simulink library "aausat3_lib"  (Simulink 8.3)
settings: Solver=ode45  StartTime=0.0  StopTime=10.0  RelTol=1e-3
undefined symbols (not defined in the file or in its folder): A_wire_mt, albedo_wrapper, alpha_0_mt, bias_gyro, bias_mag, bias_sun, Cd, coil_dim, Dim, f_sample, G, heading_gyro, heading_mag, M_earth, M_moon, M_sun, magnitude, n_mt, noise_gyro, noise_mag, noise_sun, nr_sample_sun, otoquest, otoquest_with_pro, q_method, qmethod, redfac, refldata, s_freq_gyro, s_freq_mag, s_freq_sun, sigma_0_mt, solar_absorb_coeff, solar_m_flux, SVD_method, T_0_mt, theta_e, tilt_gyro, tilt_mag, Ts
undefined symbols (not defined in the file): Actuator_Duty_Cycle_coil, Actuator_Frequency_coil, Dimensions_coil, mean_refl, Number_of_Windings_coil, rho, sim_par, svd_weigth, Wire_Cross_Sectional_Area_coil, Wire_Resistivity_Base_Temperature_coil, Wire_Resistivity_coil, Wire_Resistivity_Temperature_Coefficient_coil
libraries: aausat3_lib x118, simulink_extras x3
(part 3 of 4)

== system aausat3_lib/Orbit and Ephemeris/SGP4 position ==
  JD : Inport
  TLE : Inport  Port=2
  Enable : EnablePort
  " S-Function" : S-Function  FunctionName=sgp4S  EnableBusSupport=off
  Demux : Demux  Outputs=12
  Demux1 : Demux  Outputs=[3 3]
  JD to Minutes : Gain  Gain=1440
  Mux : Mux  Inputs=2
  Mux1 : Mux  Inputs=12
  Sum : Sum  Inputs=-+|  SaturateOnIntegerOverflow=on  InputSameDT=on  OutDataTypeStr=Inherit: Same as first input
  "TLE -> JD converter" : aausat3_lib/Other Model Utilities/TLE -> JD converter  SystemSampleTime=-1
  "km -> m" : Gain  Gain=1000  SaturateOnIntegerOverflow=on  OutDataTypeStr=Inherit: Same as input  ParamDataTypeStr=Inherit: Same as input
  "km/s -> m/s" : Gain  Gain=1000  SaturateOnIntegerOverflow=on  OutDataTypeStr=Inherit: Same as input  ParamDataTypeStr=Inherit: Same as input
  Position (I) : Outport  InitialOutput=0
  Velocity (I) : Outport  Port=2  InitialOutput=0
  wires:
  JD/1 -> Sum/2
  "km -> m"/1 -> Position (I)/1
  "km/s -> m/s"/1 -> Velocity (I)/1
  Mux/1 -> " S-Function"/1
  " S-Function"/1 -> Demux1/1
  Demux1/2 -> "km/s -> m/s"/1
  Demux1/1 -> "km -> m"/1
  TLE/1 -> Demux/1
  Demux/2 -> Mux1/2
  Demux/3 -> Mux1/3
  Demux/4 -> Mux1/4
  Demux/5 -> Mux1/5
  Demux/6 -> Mux1/6
  Demux/7 -> Mux1/7
  Demux/8 -> Mux1/8
  Demux/9 -> Mux1/9
  Demux/10 -> Mux1/10
  Demux/11 -> Mux1/11
  Demux/12 -> Mux1/12
  Mux1/1 -> Mux/2
  Demux/1 -> "TLE -> JD converter"/1
  "TLE -> JD converter"/1 -> Mux1/1, Sum/1
  Sum/1 -> JD to Minutes/1
  JD to Minutes/1 -> Mux/1

== system aausat3_lib/Orbit and Ephemeris/TLE AAUSAT-II ==
  "Constant " : Constant  Value=[JulianDay,xndt2o,xndd6o,0,bstar,0,xincl,xnodeo,eo,omegao,xmo,xno]
  "TLE " : Outport
  wires:
  "Constant "/1 -> "TLE "/1

== system aausat3_lib/Orbit and Ephemeris/TLE Orsted ==
  "Constant " : Constant  Value=[JulianDay,xndt2o,xndd6o,0,bstar,0,xincl,xnodeo,eo,omegao,xmo,xno]
  "TLE " : Outport
  wires:
  "Constant "/1 -> "TLE "/1

== system aausat3_lib/Other Model Utilities/AAUSAT-II Animation ==
  SC position : Inport
  SC quaternion : Inport  Port=2
  SC veloc : Inport  Port=3
  sun vector(I) : Inport  Port=4
  Earth rotation : Inport  Port=5
  Mux3 : Mux  Inputs=5
  S-Function : S-Function  FunctionName=aausatanim  Parameters=Config  EnableBusSupport=off
  wires:
  SC veloc/1 -> Mux3/3
  Earth rotation/1 -> Mux3/5
  sun vector(I)/1 -> Mux3/4
  SC quaternion/1 -> Mux3/2
  SC position/1 -> Mux3/1
  Mux3/1 -> S-Function/1

== system aausat3_lib/Other Model Utilities/Exposed area ==
  quaternion : Inport
  vector : Inport  Port=2
  Product2 : Product  Multiplication=Matrix(*)  RndMeth=Zero
  Product3 : Product  Multiplication=Matrix(*)  RndMeth=Zero
  Product4 : Product  Multiplication=Matrix(*)  RndMeth=Zero
  Projection Matrix1 : Subsystem
  Satellite Area : aausat3_lib/Other Model Utilities/Satellite Area  SystemSampleTime=-1
  To unit vector : aausat3_lib/Math Utilities/Vector operations/To unit vector  SystemSampleTime=-1
  Vector rotation by q : aausat3_lib/Math Utilities/Quaternion operations/Vector rotation by q  SystemSampleTime=-1
  x : Constant  Value=[dim_sat_area(1) 0 0]'
  y : Constant  Value=[0 dim_sat_area(2) 0]'
  z : Constant  Value=[0 0 dim_sat_area(3)]'
  exposed area : Outport
  wires:
  To unit vector/1 -> Vector rotation by q/2
  vector/1 -> To unit vector/1
  quaternion/1 -> Vector rotation by q/1
  Projection Matrix1/1(P matrix) -> Product2/1, Product4/1, Product3/1
  x/1 -> Product2/2
  y/1 -> Product4/2
  z/1 -> Product3/2
  Product2/1 -> Satellite Area/1
  Product4/1 -> Satellite Area/2
  Product3/1 -> Satellite Area/3
  Vector rotation by q/1 -> Projection Matrix1/1(n-vector)
  Satellite Area/1 -> exposed area/1

== system aausat3_lib/Other Model Utilities/Geocentric to  Geodetic Latitude ==
  lambda : Inport
  dist to body : Inport  Port=2
  Constant : Constant  Value=R
  Constant1 : Constant  Value=R
  Gain : Gain  Gain=pi/180
  Gain1 : Gain  Gain=180/pi
  Sum1 : Sum  Inputs=|-+
  Trigonometric Function : Trigonometry  Operator=tan
  alt : Subsystem
  delt_mu : Subsystem
  delta_lambda : Subsystem
  denom : Subsystem
  e : Subsystem
  e^4 : Subsystem
  l_point : Subsystem
  mu_alpha : Subsystem
  r_alpha : Subsystem
  rho_alpha : Subsystem
  square e : Subsystem
  square e1 : Subsystem
  x_alpha : Subsystem
  mu : Outport
  wires:
  Gain1/1 -> mu/1
  Gain/1 -> Trigonometric Function/1, mu_alpha/4(lambda), delta_lambda/2(lambda), r_alpha/1(lambda)
  dist to body/1 -> l_point/1(dist to body)
  lambda/1 -> Gain/1
  e/1(e) -> square e/1(e), x_alpha/3(e), e^4/1(e), mu_alpha/3(e)
  square e/1(e^2) -> x_alpha/4(e^2)
  Constant/1 -> square e1/1(R), x_alpha/1(R)
  square e1/1(R^2) -> mu_alpha/1(R^2)
  mu_alpha/1(mu_alpha) -> delta_lambda/1(mu_alpha), denom/1(mu_alpha), Sum1/2
  x_alpha/1(x_alpha) -> mu_alpha/2(x_alpha), r_alpha/2(x_alpha)
  Trigonometric Function/1 -> x_alpha/2(t_lat)  "t_lat"
  r_alpha/1(r_alpha) -> l_point/2(r_alpha)
  delta_lambda/1(delta_lambda) -> alt/2(delta_lambda), delt_mu/3(delta_lambda)
  l_point/1(l_point) -> alt/1(l_point), delt_mu/1(l_point)
  e^4/1(eps) -> denom/2(eps), rho_alpha/3(eps)
  denom/1(denom) -> rho_alpha/2(denom)
  alt/1(alt) -> delt_mu/2(alt)
  rho_alpha/1(rho_alpha) -> delt_mu/4(rho_alpha)
  delt_mu/1(delt_mu) -> Sum1/1
  Sum1/1 -> Gain1/1
  Constant1/1 -> rho_alpha/1(R)

== system aausat3_lib/Other Model Utilities/Geodetic to  Geocentric Latitude ==
  mu : Inport
  h : Inport  Port=2
  Constant : Constant  Value=F
  Demux : Demux  Outputs=2
  Mux : Mux  Inputs=2
  Mux1 : Mux  Inputs=2
  Product1 : Product  RndMeth=Zero
  Product2 : Product  Inputs=3  RndMeth=Zero
  Product3 : Product  RndMeth=Zero
  Radius at Geocentric Latitude : Subsystem  mask(Radius at Geocentric Latitude){units=Metric (MKS), ptype=Custom, F=F, R=R}
      mask prompts: ptype "Planet model:"; F "Flattening:"; R "Equatorial radius of planet:"
      mask help: Estimate radius of ellipsoid planet at geocentric latitude.
      mask init:
      | aeroicon('aeroblklla')
      mask Help: eval('asbhelp');
      mask TypeOptions units: Metric (MKS) | English
      mask TypeOptions ptype: Custom | Earth (WGS84)
      mask Callback ptype: aeroicon('aeroblklla')
      mask Display:
      | port_label('input',1,'\lambda_s','texmode','on')
      | port_label('output',1,'r_s','texmode','on')
  Sum : Sum  Inputs=-+
  Sum1 : Sum  Inputs=|++
  Trigonometric Function1 : Trigonometry  Operator=tan
  Trigonometric Function2 : Trigonometry  Operator=atan2
  Trigonometric Function3 : Trigonometry  Operator=atan2
  f : Constant
  rad->deg : Gain  Gain=180/pi
  rad->deg1 : Gain  Gain=180/pi
  sincos : Trigonometry  Operator=sincos
  sincos1 : Trigonometry  Operator=sincos
  lambda : Outport
  wires:
  rad->deg1/1 -> Radius at Geocentric Latitude/1(lambda_s)
  mu/1 -> sincos1/1, Trigonometric Function1/1
  Constant/1 -> Sum/1
  f/1 -> Trigonometric Function2/2, Sum/2
  Product2/1 -> Trigonometric Function2/1
  Sum/1 -> Product2/3, Product2/2
  Trigonometric Function2/1 -> sincos/1, rad->deg1/1
  Trigonometric Function1/1 -> Product2/1
  Radius at Geocentric Latitude/1(r_s) -> Product1/1
  rad->deg/1 -> lambda/1
  sincos1/1 -> Mux/1
  h/1 -> Product3/1
  sincos1/2 -> Mux/2
  sincos/1 -> Mux1/1
  sincos/2 -> Mux1/2
  Mux/1 -> Product3/2
  Mux1/1 -> Product1/2
  Product3/1 -> Sum1/1
  Product1/1 -> Sum1/2
  Trigonometric Function3/1 -> rad->deg/1
  Sum1/1 -> Demux/1
  Demux/1 -> Trigonometric Function3/1
  Demux/2 -> Trigonometric Function3/2

== system aausat3_lib/Other Model Utilities/Randome 3D Vector ==
  Demux : Demux  Outputs=3
  Divide : Product  Inputs=*/
  Math Function : Math  Operator=square  SaturateOnIntegerOverflow=on
  Math Function1 : Math  Operator=square  SaturateOnIntegerOverflow=on
  Math Function2 : Math  Operator=square  SaturateOnIntegerOverflow=on
  Math Function3 : Math  Operator=sqrt  SaturateOnIntegerOverflow=on
  Random Number : RandomNumber  Mean=mean  Variance=[var,0,0]  Seed=seed(1)
  Random Number1 : RandomNumber  Mean=mean  Variance=[0,var,0]  Seed=seed(2)
  Random Number2 : RandomNumber  Mean=mean  Variance=[0,0,var]  Seed=seed(3)
  Sum : Sum  Inputs=+++
  Sum1 : Sum  Inputs=+++
  Sum2 : Sum  Inputs=+++
  Rand_vec : Outport
  wires:
  Divide/1 -> Rand_vec/1
  Sum2/1 -> Math Function3/1
  Demux/3 -> Sum2/3
  Demux/2 -> Sum2/2
  Demux/1 -> Sum2/1
  Sum/1 -> Demux/1
  Sum1/1 -> Divide/1
  Math Function3/1 -> Divide/2
  Random Number2/1 -> Sum1/3, Math Function2/1
  Random Number1/1 -> Sum1/2, Math Function1/1
  Random Number/1 -> Sum1/1, Math Function/1
  Math Function2/1 -> Sum/3
  Math Function1/1 -> Sum/2
  Math Function/1 -> Sum/1

== system aausat3_lib/Other Model Utilities/SC ECI to geodetic position converter ==
  Simulation time  t(JD) : Inport
  Spacecraft position R_sc(I) : Inport  Port=2
  Cartesian to Spherical : simulink_extras/Transformations/Cartesian to Spherical  SystemSampleTime=-1
  Demux1 : Demux  Outputs=3
  ECI->ECEF quaternion : aausat3_lib/Orbit and Ephemeris/ECI->ECEF quaternion  SystemSampleTime=-1
  Earth radius WGS84 : Fcn  Expr=sqrt(((a^2*cos(u(1)))^2+(b^2*sin(u(1)))^2)/((a*cos(u(1)))^2+(b*sin(u(1)))^2))
  Eccentricity : Constant  Value=sqrt(a^2-b^2)/a
  Geocentric to  Geodetic Latitude : aausat3_lib/Other Model Utilities/Geocentric to  Geodetic Latitude  SystemSampleTime=-1
  Geodetic elevation : Fcn  Expr=(u(4)*cos(pi/180*u(3)-pi/180*u(5))-1/u(1))/1000-u(2)
  Mux : Mux  Inputs=2
  Mux1 : Mux  Inputs=5
  N : Fcn  Expr=(1-u(1)^2*sin(u(2))^2)^(-1/2)
  Vector rotation by q : aausat3_lib/Math Utilities/Quaternion operations/Vector rotation by q  SystemSampleTime=-1
  convert to  geocentric latitude : Fcn  Expr=(90-180/pi*u(1))
  convert to  geocentric longitude : Fcn  Expr=180/pi*u(1)
  Geodetic elevation (km) : Outport
  Geodetic longitude  (degree) : Outport  Port=2
  Geodetic latitude  (degree) : Outport  Port=3
  wires:
  Spacecraft position R_sc(I)/1 -> Vector rotation by q/2
  Vector rotation by q/1 -> Demux1/1
  Demux1/1 -> Cartesian to Spherical/1
  Demux1/2 -> Cartesian to Spherical/2
  Demux1/3 -> Cartesian to Spherical/3
  Cartesian to Spherical/1 -> Geocentric to  Geodetic Latitude/2, Mux1/4
  Cartesian to Spherical/2 -> convert to  geocentric longitude/1
  Cartesian to Spherical/3 -> convert to  geocentric latitude/1
  Simulation time  t(JD)/1 -> ECI->ECEF quaternion/1
  ECI->ECEF quaternion/1 -> Vector rotation by q/1
  convert to  geocentric latitude/1 -> Geocentric to  Geodetic Latitude/1, Mux1/5
  convert to  geocentric longitude/1 -> Geodetic longitude  (degree)/1
  Geocentric to  Geodetic Latitude/1 -> Geodetic latitude  (degree)/1, Earth radius WGS84/1, Mux/2, Mux1/3
  Mux/1 -> N/1
  Eccentricity/1 -> Mux/1
  Mux1/1 -> Geodetic elevation/1
  Earth radius WGS84/1 -> Mux1/2
  N/1 -> Mux1/1
  Geodetic elevation/1 -> Geodetic elevation (km)/1

== system aausat3_lib/Other Model Utilities/Satellite Area ==
  px : Inport
  py : Inport  Port=2
  pz : Inport  Port=3
  Cross Product : aausat3_lib/Math Utilities/Vector operations/Cross Product  SystemSampleTime=-1
  Cross Product1 : aausat3_lib/Math Utilities/Vector operations/Cross Product  SystemSampleTime=-1
  Cross Product2 : aausat3_lib/Math Utilities/Vector operations/Cross Product  SystemSampleTime=-1
  Dot Product : DotProduct  InputSameDT=on  OutDataTypeStr=Inherit: Inherit via internal rule
  Dot Product1 : DotProduct  InputSameDT=on  OutDataTypeStr=Inherit: Inherit via internal rule
  Dot Product2 : DotProduct  InputSameDT=on  OutDataTypeStr=Inherit: Inherit via internal rule
  Sum : Sum  Inputs=+|+|+
  inv1 : Math  Operator=sqrt  SaturateOnIntegerOverflow=on
  inv2 : Math  Operator=sqrt  SaturateOnIntegerOverflow=on
  inv3 : Math  Operator=sqrt  SaturateOnIntegerOverflow=on
  area_sat : Outport
  wires:
  Dot Product/1 -> inv1/1
  Cross Product/1 -> Dot Product/2, Dot Product/1
  px/1 -> Cross Product/1, Cross Product1/1
  inv1/1 -> Sum/1
  py/1 -> Cross Product/2, Cross Product2/1
  Dot Product1/1 -> inv2/1
  Cross Product1/1 -> Dot Product1/1, Dot Product1/2
  Dot Product2/1 -> inv3/1
  Cross Product2/1 -> Dot Product2/2, Dot Product2/1
  pz/1 -> Cross Product1/2, Cross Product2/2
  inv2/1 -> Sum/2
  inv3/1 -> Sum/3
  Sum/1 -> area_sat/1

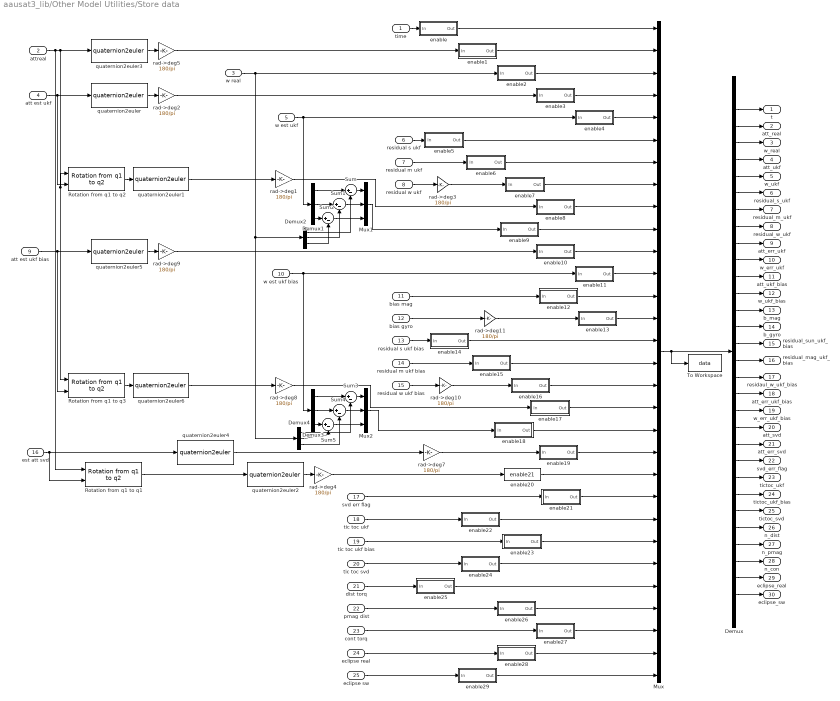
== system aausat3_lib/Other Model Utilities/Store data ==
  time : Inport
  attreal : Inport  Port=2
  w real : Inport  Port=3
  att est ukf : Inport  Port=4
  w est ukf : Inport  Port=5
  residual s ukf : Inport  Port=6
  residual m ukf : Inport  Port=7
  residual w ukf : Inport  Port=8
  att est ukf bias : Inport  Port=9
  w est ukf bias : Inport  Port=10
  bias mag : Inport  Port=11
  bias gyro : Inport  Port=12
  residual s ukf bias : Inport  Port=13
  residual m ukf bias : Inport  Port=14
  residual w ukf bias : Inport  Port=15
  est att svd : Inport  Port=16
  svd err flag : Inport  Port=17
  tic toc ukf : Inport  Port=18
  tic toc ukf bias : Inport  Port=19
  tic toc svd : Inport  Port=20
  dist torq : Inport  Port=21
  pmag dist : Inport  Port=22
  cont torq : Inport  Port=23
  eclipse real : Inport  Port=24
  eclipse sw : Inport  Port=25
  Demux : Demux  Outputs=30
  Demux{1..4} (4 alike) : Demux  Outputs=3
  Mux : Mux  Inputs=30
  Mux1 : Mux  Inputs=3
  Mux2 : Mux  Inputs=3
  Rotation from q1 to q1 : aausat3_lib/Math Utilities/Quaternion operations/Rotation from q1 to q2  SystemSampleTime=-1
  Rotation from q1 to q2 : aausat3_lib/Math Utilities/Quaternion operations/Rotation from q1 to q2  SystemSampleTime=-1
  Rotation from q1 to q3 : aausat3_lib/Math Utilities/Quaternion operations/Rotation from q1 to q2  SystemSampleTime=-1
  Sum{,1..5} (6 alike) : Sum  Inputs=|+-
  To Workspace : ToWorkspace  VariableName=data  SampleTime=1/f_sample
  enable : Subsystem  mask{enable_signal=enable_t}
      mask prompts: enable_signal "Signal name:"
  enable1 : Subsystem  mask{enable_signal=enable_att}
      mask prompts: enable_signal "Signal name:"
  enable10 : Subsystem  mask{enable_signal=enable_att_ukf_bias}
      mask prompts: enable_signal "Signal name:"
  enable11 : Subsystem  mask{enable_signal=enable_w_ukf_bias}
      mask prompts: enable_signal "Signal name:"
  enable12 : Subsystem  mask{enable_signal=enable_b_mag}
      mask prompts: enable_signal "Signal name:"
  enable13 : Subsystem  mask{enable_signal=enable_b_gyro}
      mask prompts: enable_signal "Signal name:"
  enable14 : Subsystem  mask{enable_signal=enable_r_sun_ukf_bias}
      mask prompts: enable_signal "Signal name:"
  enable15 : Subsystem  mask{enable_signal=enable_r_mag_ukf_bias}
      mask prompts: enable_signal "Signal name:"
  enable16 : Subsystem  mask{enable_signal=enable_r_w_ukf_bias}
      mask prompts: enable_signal "Signal name:"
  enable17 : Subsystem  mask{enable_signal=enable_eia_ukf_bias}
      mask prompts: enable_signal "Signal name:"
  enable18 : Subsystem  mask{enable_signal=enable_eiw_ukf_bias}
      mask prompts: enable_signal "Signal name:"
  enable19 : Subsystem  mask{enable_signal=enable_att_svd}
      mask prompts: enable_signal "Signal name:"
  enable2 : Subsystem  mask{enable_signal=enable_w}
      mask prompts: enable_signal "Signal name:"
  enable20 : aausat3_lib/Other Model Utilities/Store data/enable21  SystemSampleTime=-1  enable_signal=enable_svd_att_err
  enable21 : Subsystem  mask{enable_signal=enable_svd_err}
      mask prompts: enable_signal "Signal name:"
  enable22 : Subsystem  mask{enable_signal=enable_tictoc}
      mask prompts: enable_signal "Signal name:"
  enable23 : Subsystem  mask{enable_signal=enable_tictoc_ukf_bias}
      mask prompts: enable_signal "Signal name:"
  enable24 : Subsystem  mask{enable_signal=enable_tictoc_svd}
      mask prompts: enable_signal "Signal name:"
  enable25 : Subsystem  mask{enable_signal=enable_n_dist}
      mask prompts: enable_signal "Signal name:"
  enable26 : Subsystem  mask{enable_signal=enable_n_pmag}
      mask prompts: enable_signal "Signal name:"
  enable27 : Subsystem  mask{enable_signal=enable_n_con}
      mask prompts: enable_signal "Signal name:"
  enable28 : Subsystem  mask{enable_signal=enable_eclip_real}
      mask prompts: enable_signal "Signal name:"
  enable29 : Subsystem  mask{enable_signal=enable_eclip_sw}
      mask prompts: enable_signal "Signal name:"
  enable3 : Subsystem  mask{enable_signal=enable_att_ukf}
      mask prompts: enable_signal "Signal name:"
  enable4 : Subsystem  mask{enable_signal=enable_w_ukf}
      mask prompts: enable_signal "Signal name:"
  enable5 : Subsystem  mask{enable_signal=enable_r_sun}
      mask prompts: enable_signal "Signal name:"
  enable6 : Subsystem  mask{enable_signal=enable_r_mag}
      mask prompts: enable_signal "Signal name:"
  enable7 : Subsystem  mask{enable_signal=enable_r_w}
      mask prompts: enable_signal "Signal name:"
  enable8 : Subsystem  mask{enable_signal=enable_eia}
      mask prompts: enable_signal "Signal name:"
  enable9 : Subsystem  mask{enable_signal=enable_eiw}
      mask prompts: enable_signal "Signal name:"
  quaternion2euler{,1..6} (7 alike) : aausat3_lib/Math Utilities/Quaternion operations/quaternion2euler  SystemSampleTime=-1
  rad->deg{1..5,7..11} (10 alike) : Gain  Gain=180/pi
  t : Outport
  att_real : Outport  Port=2
  w_real : Outport  Port=3
  att_ukf : Outport  Port=4
  w_ukf : Outport  Port=5
  residual_s_ukf : Outport  Port=6
  residual_m_ukf : Outport  Port=7
  residual_w_ukf : Outport  Port=8
  att_err_ukf : Outport  Port=9
  w_err_ukf : Outport  Port=10
  att_ukf_bias : Outport  Port=11
  w_ukf_bias : Outport  Port=12
  b_mag : Outport  Port=13
  b_gyro : Outport  Port=14
  residual_sun_ukf_bias : Outport  Port=15
  residual_mag_ukf_bias : Outport  Port=16
  residaul_w_ukf_bias : Outport  Port=17
  att_err_ukf_bias : Outport  Port=18
  w_err_ukf_bias : Outport  Port=19
  att_svd : Outport  Port=20
  att_err_svd : Outport  Port=21
  svd_err_flag : Outport  Port=22
  tictoc_ukf : Outport  Port=23
  tictoc_ukf_bias : Outport  Port=24
  tictoc_svd : Outport  Port=25
  n_dist : Outport  Port=26
  n_pmag : Outport  Port=27
  n_con : Outport  Port=28
  eclipse_real : Outport  Port=29
  eclipse_sw : Outport  Port=30
  wires:
  Demux/22 -> svd_err_flag/1
  Demux/25 -> tictoc_svd/1
  Demux/26 -> n_dist/1
  Demux/30 -> eclipse_sw/1
  Demux/29 -> eclipse_real/1
  Demux/28 -> n_con/1
  Demux/27 -> n_pmag/1
  Demux/24 -> tictoc_ukf_bias/1
  Demux/23 -> tictoc_ukf/1
  enable21/1(Out) -> Mux/22
  svd err flag/1 -> enable21/1(In)
  enable24/1(Out) -> Mux/25
  tic toc svd/1 -> enable24/1(In)
  enable29/1(Out) -> Mux/30
  eclipse sw/1 -> enable29/1(In)
  enable25/1(Out) -> Mux/26
  enable26/1(Out) -> Mux/27
  enable28/1(Out) -> Mux/29
  dist torq/1 -> enable25/1(In)
  pmag dist/1 -> enable26/1(In)
  cont torq/1 -> enable27/1(In)
  eclipse real/1 -> enable28/1(In)
  enable23/1(Out) -> Mux/24
  tic toc ukf bias/1 -> enable23/1(In)
  enable22/1(Out) -> Mux/23
  tic toc ukf/1 -> enable22/1(In)
  enable27/1(Out) -> Mux/28
  Demux/21 -> att_err_svd/1
  Demux/20 -> att_svd/1
  Demux/19 -> w_err_ukf_bias/1
  Demux/18 -> att_err_ukf_bias/1
  Demux/17 -> residaul_w_ukf_bias/1
  Demux/16 -> residual_mag_ukf_bias/1
  Demux/15 -> residual_sun_ukf_bias/1
  Demux/14 -> b_gyro/1
  Demux/13 -> b_mag/1
  Demux/12 -> w_ukf_bias/1
  Demux/11 -> att_ukf_bias/1
  Demux/10 -> w_err_ukf/1
  Demux/9 -> att_err_ukf/1
  Demux/8 -> residual_w_ukf/1
  Demux/7 -> residual_m_ukf/1
  Demux/6 -> residual_s_ukf/1
  Demux/5 -> w_ukf/1
  Demux/4 -> att_ukf/1
  Demux/3 -> w_real/1
  Demux/2 -> att_real/1
  Demux/1 -> t/1
  enable5/1(Out) -> Mux/6
  enable6/1(Out) -> Mux/7
  enable7/1(Out) -> Mux/8
  enable8/1(Out) -> Mux/9
  enable9/1(Out) -> Mux/10
  enable10/1(Out) -> Mux/11
  enable11/1(Out) -> Mux/12
  enable12/1(Out) -> Mux/13
  enable13/1(Out) -> Mux/14
  enable15/1(Out) -> Mux/16
  enable14/1(Out) -> Mux/15
  enable16/1(Out) -> Mux/17
  enable17/1(Out) -> Mux/18
  enable18/1(Out) -> Mux/19
  enable19/1(Out) -> Mux/20
  Demux4/3 -> Sum4/2
  Demux4/2 -> Sum5/2
  enable20/1 -> Mux/21
  enable4/1(Out) -> Mux/5
  enable3/1(Out) -> Mux/4
  enable2/1(Out) -> Mux/3
  enable1/1(Out) -> Mux/2
  enable/1(Out) -> Mux/1
  residual s ukf bias/1 -> enable14/1(In)
  w est ukf bias/1 -> enable11/1(In), Demux3/1
  bias mag/1 -> enable12/1(In)
  residual m ukf bias/1 -> enable15/1(In)
  Demux3/3 -> Sum5/1
  Demux4/1 -> Sum3/2
  Sum4/1 -> Mux2/2
  Sum5/1 -> Mux2/3
  Sum3/1 -> Mux2/1
  Demux3/2 -> Sum4/1
  Demux3/1 -> Sum3/1
  bias gyro/1 -> rad->deg11/1
  rad->deg11/1 -> enable13/1(In)
  quaternion2euler6/1 -> rad->deg8/1
  quaternion2euler5/1 -> rad->deg9/1
  att est ukf bias/1 -> Rotation from q1 to q3/2, quaternion2euler5/1
  Rotation from q1 to q3/1 -> quaternion2euler6/1
  residual w ukf bias/1 -> rad->deg10/1
  rad->deg10/1 -> enable16/1(In)
  rad->deg9/1 -> enable10/1(In)
  rad->deg8/1 -> enable17/1(In)
  Mux2/1 -> enable18/1(In)
  rad->deg7/1 -> enable19/1(In)
  quaternion2euler4/1 -> rad->deg7/1
  Mux/1 -> To Workspace/1, Demux/1
  time/1 -> enable/1(In)
  w real/1 -> Demux4/1, Demux2/1, enable2/1(In)
  w est ukf/1 -> enable4/1(In), Demux1/1
  residual s ukf/1 -> enable5/1(In)
  residual m ukf/1 -> enable6/1(In)
  est att svd/1 -> quaternion2euler4/1, Rotation from q1 to q1/2
  Demux1/3 -> Sum2/1
  Demux2/3 -> Sum2/2
  Demux2/2 -> Sum1/2
  Demux2/1 -> Sum/2
  Sum1/1 -> Mux1/2
  Sum2/1 -> Mux1/3
  Sum/1 -> Mux1/1
  Demux1/2 -> Sum1/1
  Demux1/1 -> Sum/1
  quaternion2euler2/1 -> rad->deg4/1
  Rotation from q1 to q1/1 -> quaternion2euler2/1
  quaternion2euler3/1 -> rad->deg5/1
  attreal/1 -> Rotation from q1 to q3/1, Rotation from q1 to q2/1, quaternion2euler3/1, Rotation from q1 to q1/1
  quaternion2euler1/1 -> rad->deg1/1
  quaternion2euler/1 -> rad->deg2/1
  att est ukf/1 -> Rotation from q1 to q2/2, quaternion2euler/1
  Rotation from q1 to q2/1 -> quaternion2euler1/1
  rad->deg5/1 -> enable1/1(In)
  residual w ukf/1 -> rad->deg3/1
  rad->deg3/1 -> enable7/1(In)
  rad->deg2/1 -> enable3/1(In)
  rad->deg1/1 -> enable8/1(In)
  Mux1/1 -> enable9/1(In)
  rad->deg4/1 -> enable20/1

== system aausat3_lib/Other Model Utilities/TLE -> JD converter ==
  TLE (Epoch time) : Inport
  Add century : Constant  Value=1900
  Add century1 : Constant  Value=2000
  Gain1 : Gain  Gain=1/1000
  Gain2 : Gain  Gain=1/1000
  Gain3 : Gain  Gain=1000
  Sum1 : Sum  Inputs=++|
  Sum3 : Sum  Inputs=++|
  Sum4 : Sum  Inputs=++-
  Sum5 : Sum  Inputs=|+-
  calculate JD for given year  at 1. jan time 00.00 : Fcn  Expr=367*u(1)-floor(7*(u(1)+floor((1+9)/12))/4)+floor(275*1/9)+1+1721013.5+0/24
  extract year : Rounding
  substract 1 day : Constant
  year 1950-1999 or  2000-2049? : Switch  Threshold=50
  JD : Outport
  wires:
  Add century/1 -> Sum3/1
  Gain2/1 -> Sum3/2, year 1950-1999 or  2000-2049?/2
  TLE (Epoch time)/1 -> Gain2/1, Gain1/1
  extract year/1 -> Sum5/2, calculate JD for given year  at 1. jan time 00.00/1
  calculate JD for given year  at 1. jan time 00.00/1 -> Sum4/2
  Sum5/1 -> Gain3/1
  Sum4/1 -> JD/1
  Gain3/1 -> Sum4/1
  substract 1 day/1 -> Sum4/3
  Add century1/1 -> Sum1/1
  Gain1/1 -> Sum1/2
  year 1950-1999 or  2000-2049?/1 -> extract year/1, Sum5/1
  Sum1/1 -> year 1950-1999 or  2000-2049?/3
  Sum3/1 -> year 1950-1999 or  2000-2049?/1

== system aausat3_lib/Sensor Emulation/Gyroscopes ==
  Omega_S : Inport
  Bias1 : Constant  Value=bias_gyro
  Cartesian to Spherical : aausat3_lib/Sensor Emulation/Sun sensors/Cartesian to Spherical  SystemSampleTime=-1
  Demux1 : Demux  Outputs=3
  Demux2 : Demux  Outputs=3
  Demux3 : Demux  Outputs=3
  Mux1 : Mux  Inputs=3
  Mux2 : Mux  Inputs=3
  Noise1 : RandomNumber  Variance=((pi/180)*noise_gyro)^2  Seed=1  SampleTime=0.1
  Noise2 : RandomNumber  Variance=((pi/180)*noise_gyro)^2  Seed=999  SampleTime=0.1
  Noise3 : RandomNumber  Variance=((pi/180)*noise_gyro)^2  Seed=46945  SampleTime=0.1
  Spherical to Cartesian : aausat3_lib/Sensor Emulation/Sun sensors/Spherical to Cartesian  SystemSampleTime=-1
  Sum1 : Sum  Inputs=|++
  Sum3 : Sum  Inputs=+++
  Sum6 : Sum  Inputs=+++
  Sum7 : Sum  Inputs=+++
  Sum8 : Sum  Inputs=|++
  Zero-Order Hold : ZeroOrderHold  SampleTime=1/s_freq_gyro
  "deg -> rad" : Gain  Gain=pi/180
  "deg -> rad1" : Gain  Gain=pi/180
  "deg -> rad2" : Gain  Gain=pi/180
  displacement : Constant  Value=heading_gyro
  displacement1 : Constant  Value=tilt_gyro
  Omega_S_meas : Outport
  wires:
  Noise1/1 -> Sum6/3
  "deg -> rad2"/1 -> Sum8/2
  displacement1/1 -> "deg -> rad2"/1
  "deg -> rad1"/1 -> Sum1/2
  displacement/1 -> "deg -> rad1"/1
  "deg -> rad"/1 -> Demux3/1
  Bias1/1 -> "deg -> rad"/1
  Noise2/1 -> Sum7/3
  Noise3/1 -> Sum3/3
  Zero-Order Hold/1 -> Omega_S_meas/1
  Omega_S/1 -> Demux1/1
  Demux1/3 -> Sum3/2
  Demux1/2 -> Sum7/2
  Demux1/1 -> Sum6/2
  Sum3/1 -> Mux1/3
  Sum7/1 -> Mux1/2
  Sum6/1 -> Mux1/1
  Demux2/1 -> Cartesian to Spherical/1
  Demux2/2 -> Cartesian to Spherical/2
  Demux2/3 -> Cartesian to Spherical/3
  Spherical to Cartesian/1 -> Mux2/1
  Spherical to Cartesian/2 -> Mux2/2
  Spherical to Cartesian/3 -> Mux2/3
  Cartesian to Spherical/1 -> Spherical to Cartesian/1
  Cartesian to Spherical/2 -> Sum1/1
  Sum1/1 -> Spherical to Cartesian/2
  Sum8/1 -> Spherical to Cartesian/3
  Cartesian to Spherical/3 -> Sum8/1
  Mux1/1 -> Demux2/1
  Mux2/1 -> Zero-Order Hold/1
  Demux3/1 -> Sum6/1
  Demux3/2 -> Sum7/1
  Demux3/3 -> Sum3/1

== system aausat3_lib/Sensor Emulation/Magnetometers ==
  q_I_S : Inport
  Mag_I : Inport  Port=2
  Bias : Constant  Value=bias_mag
  Cartesian to Spherical : aausat3_lib/Sensor Emulation/Sun sensors/Cartesian to Spherical  SystemSampleTime=-1
  Demux : Demux  Outputs=3
  Demux1 : Demux  Outputs=3
  Demux2 : Demux  Outputs=3
  Mux : Mux  Inputs=3
  Mux2 : Mux  Inputs=3
  Noise1 : RandomNumber  Variance=((pi/180)*noise_mag)^2  Seed=23771  SampleTime=0.1
  Noise2 : RandomNumber  Variance=((pi/180)*noise_mag)^2  Seed=5000  SampleTime=0.1
  Spherical to Cartesian : aausat3_lib/Sensor Emulation/Sun sensors/Spherical to Cartesian  SystemSampleTime=-1
  Sum : Sum  Inputs=++|
  Sum1 : Sum  Inputs=+++
  Sum2 : Sum  Inputs=+++
  Sum4 : Sum  Inputs=++|
  Sum5 : Sum  Inputs=++|
  Vector rotation by q : Subsystem
  Zero-Order Hold : ZeroOrderHold  SampleTime=1/s_freq_mag
  "[nT] -> [T]" : Gain  Gain=10^(-9)
  "deg -> rad" : Gain  Gain=pi/180
  "deg -> rad1" : Gain  Gain=pi/180
  displacement : Constant  Value=heading_mag
  displacement1 : Constant  Value=tilt_mag
  Mag_S_meas : Outport
  wires:
  "deg -> rad"/1 -> Sum1/3
  Noise2/1 -> Sum2/1
  Noise1/1 -> Sum1/1
  Cartesian to Spherical/2 -> Sum1/2
  "[nT] -> [T]"/1 -> Demux1/1
  Bias/1 -> "[nT] -> [T]"/1
  "deg -> rad1"/1 -> Sum2/3
  displacement1/1 -> "deg -> rad1"/1
  displacement/1 -> "deg -> rad"/1
  q_I_S/1 -> Vector rotation by q/1(q)
  Mag_I/1 -> Vector rotation by q/2(V)
  Vector rotation by q/1(q'Vq) -> Demux/1
  Sum4/1 -> Mux/1
  Sum5/1 -> Mux/2
  Sum/1 -> Mux/3
  Demux/1 -> Sum4/2
  Demux/2 -> Sum5/2
  Demux/3 -> Sum/2
  Zero-Order Hold/1 -> Mag_S_meas/1
  Demux2/1 -> Cartesian to Spherical/1
  Demux2/2 -> Cartesian to Spherical/2
  Demux2/3 -> Cartesian to Spherical/3
  Spherical to Cartesian/1 -> Mux2/1
  Spherical to Cartesian/2 -> Mux2/2
  Spherical to Cartesian/3 -> Mux2/3
  Cartesian to Spherical/1 -> Spherical to Cartesian/1
  Sum1/1 -> Spherical to Cartesian/2
  Sum2/1 -> Spherical to Cartesian/3
  Cartesian to Spherical/3 -> Sum2/2
  Mux/1 -> Demux2/1
  Mux2/1 -> Zero-Order Hold/1
  Demux1/1 -> Sum4/1
  Demux1/2 -> Sum5/1
  Demux1/3 -> Sum/1

== system aausat3_lib/Sensor Emulation/Measurements ==
  q_I_S : Inport
  Mag_I : Inport  Port=2
  Omega_S : Inport  Port=3
  Pos_Sun_I : Inport  Port=4
  Eclipse : Inport  Port=5
  Gyroscopes : aausat3_lib/Sensor Emulation/Gyroscopes  SystemSampleTime=-1  s_freq_gyro=s_freq_gyro  noise_gyro=noise_gyro  bias_gyro=bias_gyro  heading_gyro=heading_gyro  tilt_gyro=tilt_gyro
  Magnetometers : aausat3_lib/Sensor Emulation/Magnetometers  SystemSampleTime=-1  s_freq_mag=s_freq_mag  noise_mag=noise_mag  bias_mag=bias_mag  heading_mag=heading_mag  tilt_mag=tilt_mag
  Sun sensors : aausat3_lib/Sensor Emulation/Sun sensors  SystemSampleTime=-1  s_freq_sun=s_freq_sun  noise_sun=noise_sun  bias_sun=bias_sun  nr_sample_sun=nr_sample_sun
  Sun_S_meas : Outport
  Mag_S_meas : Outport  Port=2
  Omega_S_meas : Outport  Port=3
  wires:
  q_I_S/1 -> Magnetometers/1, Sun sensors/3
  Mag_I/1 -> Magnetometers/2
  Magnetometers/1 -> Mag_S_meas/1
  Gyroscopes/1 -> Omega_S_meas/1
  Eclipse/1 -> Sun sensors/1
  Pos_Sun_I/1 -> Sun sensors/2
  Sun sensors/1 -> Sun_S_meas/1
  Omega_S/1 -> Gyroscopes/1

== system aausat3_lib/Sensor Emulation/Sun sensors ==
  Eclipse : Inport
  Pos_Sun_I : Inport  Port=2
  q_I_S : Inport  Port=3
  Bias : Constant  Value=bias_sun
  Cartesian to Spherical : Subsystem  mask(Cart2Sph){}
      mask help:
      | Transformation from cartesian to spherical coordinates.
      | [x, y, z] -> [r, theta, phi]
      |
      | p = hypot(x,y); r = hypot(p,z);
      | theta = atan(y/x);
      | phi = atan(p/z);
      mask Help: web([docroot '/toolbox/simulink/ref_extras/cartesiantospherical.html'])
      mask Display: plot(0,0,100,100,[45,40,35,40,40],[85,95,85,95,30],[22,10,14,10,40,95,85,95,85],[12,10,20,10,30,30,25,30,35],[70,40],[80,30],[54,52,50,47,44,40],[53,55,56,58,59,59])
  Constant : Constant  Value=0
  Demux1 : Demux  Outputs=2
  Demux2 : Demux  Outputs=3
  Mux2 : Mux  Inputs=3
  Noise1 : RandomNumber  Variance=((-pi/180)*noise_sun)^2  Seed=95817  SampleTime=0.1
  Noise2 : RandomNumber  Variance=((-pi/180)*noise_sun)^2  Seed=74619  SampleTime=0.1
  Pulse Generator : DiscretePulseGenerator  Period=(1/s_freq_sun)/0.1  PulseWidth=nr_sample_sun  SampleTime=0.1
  Spherical to Cartesian : Subsystem  mask(Sph2Cart){}
      mask help:
      | Transformation from spherical to cartesian coordinates.
      | [r, theta, phi] -> [x, y, z]
      |
      | x = r * sin(phi) * cos(theta);
      | y = r * sin(phi) * sin(theta);
      | z = r * cos(phi);
      mask Help: web([docroot '/toolbox/simulink/ref_extras/sphericaltocartesian.html'])
      mask Display: plot(0,0,100,100,[45,40,35,40,40],[85,95,85,95,40],[85,95,85,95,40],[35,40,45,40,40],[60,40,10,20,10,14],[70,40,10,13,10,20],[56,45],[70,70],[60,60],[50,60],[60,60],[30,40],[50,60],[20,20],[30,40],[20,20],[45,55],[35,25],[75,65],[35,25])
  Sum1 : Sum  Inputs=+++
  Sum8 : Sum  Inputs=+++
  Switch : Switch  Criteria=u2 > Threshold  Threshold=0.5  ZeroCross=off
  Switch1 : Switch  Criteria=u2 > Threshold  Threshold=0.5  ZeroCross=off
  Vector rotation by q : Subsystem
  Zero-Order Hold : ZeroOrderHold  SampleTime=1/s_freq_sun
  Zero-Order Hold1 : ZeroOrderHold  SampleTime=0.1
  "deg -> rad" : Gain  Gain=pi/180
  Sun_S_meas : Outport
  wires:
  Noise2/1 -> Sum8/3
  "deg -> rad"/1 -> Demux1/1
  Demux1/1 -> Sum1/1
  Demux1/2 -> Sum8/1
  Noise1/1 -> Sum1/3
  Mux2/1 -> Switch/3
  Vector rotation by q/1(q'Vq) -> Demux2/1
  Demux2/1 -> Cartesian to Spherical/1(x)
  Demux2/2 -> Cartesian to Spherical/2(y)
  Demux2/3 -> Cartesian to Spherical/3(z)
  Spherical to Cartesian/1(X) -> Mux2/1
  Spherical to Cartesian/2(Y) -> Mux2/2
  Spherical to Cartesian/3(Z) -> Mux2/3
  Cartesian to Spherical/1("r ") -> Spherical to Cartesian/1(r)
  Sum1/1 -> Spherical to Cartesian/2(theta)
  Sum8/1 -> Spherical to Cartesian/3(phi)
  Pos_Sun_I/1 -> Vector rotation by q/2(V)
  q_I_S/1 -> Vector rotation by q/1(q)
  Eclipse/1 -> Switch/2
  Constant/1 -> Switch/1
  Zero-Order Hold1/1 -> Switch1/1
  Zero-Order Hold/1 -> Switch1/3
  Pulse Generator/1 -> Switch1/2
  Switch1/1 -> Sun_S_meas/1
  Switch/1 -> Zero-Order Hold1/1, Zero-Order Hold/1
  Cartesian to Spherical/2(theta) -> Sum1/2
  Cartesian to Spherical/3(phi) -> Sum8/2
  Bias/1 -> "deg -> rad"/1

== system aausat3_lib/Actuator Emulation/Permanent Magnet/Vector rotation by q ==
  q : Inport
  V : Inport  Port=2
  Constant : Constant  Value=0
  Demux : Demux  Outputs=3
  Demux1 : Demux
  Mux : Mux
  Mux1 : Mux  Inputs=3
  Quaternion inverter : Subsystem
  Quaternion mulitiplication : S-Function  FunctionName=qmul  EnableBusSupport=off
  Quaternion mulitiplication1 : S-Function  FunctionName=qmul  EnableBusSupport=off
  Terminator : Terminator
  q'Vq : Outport
  wires:
  Mux1/1 -> q'Vq/1
  Demux1/4 -> Terminator/1
  Demux1/3 -> Mux1/3
  Demux1/2 -> Mux1/2
  Demux1/1 -> Mux1/1
  Quaternion mulitiplication1/1 -> Demux1/1
  Quaternion mulitiplication/1 -> Quaternion mulitiplication1/1
  Mux/1 -> Quaternion mulitiplication/2
  Constant/1 -> Mux/4
  Demux/3 -> Mux/3
  Demux/2 -> Mux/2
  Demux/1 -> Mux/1
  V/1 -> Demux/1
  Quaternion inverter/1(q^-1) -> Quaternion mulitiplication/1
  q/1 -> Quaternion mulitiplication1/2, Quaternion inverter/1(q)

== system aausat3_lib/Disturbances/Atmospheric/Density7 ==
  i : Inport
  r : Inport  Port=2
  jd : Inport  Port=3
  Add : Sum
  Constant : Constant
  Constant1 : Constant  Value=2
  Constant2 : Constant  Value=2
  Display{,1,3..4} (4 alike) : Display
  Divide : Product  Inputs=/*
  Divide1 : Product  Inputs=*/
  Embedded MATLAB Function : MATLAB Function  TreatAsAtomicUnit=on
  Exponent n Eq: [(1/22.5)*i]+2 : Subsystem
  Subsystem : Subsystem
  Unit Vector : Subsystem
  cosn(si/2) : Math  Operator=pow  SaturateOnIntegerOverflow=on
  eb.er : DotProduct  InputSameDT=on  OutDataTypeStr=Inherit: Inherit via internal rule
  rho : Outport
  geo-h : Outport  Port=2
  wires:
  jd/1 -> Subsystem/1(JD)
  Divide1/1 -> cosn(si/2)/2
  Subsystem/1(e-sun) -> eb.er/1
  Embedded MATLAB Function/2(h) -> geo-h/1, Display1/1
  Embedded MATLAB Function/1(rho) -> Display/1, rho/1
  cosn(si/2)/1 -> Display4/1, Embedded MATLAB Function/1(cosn_si2)
  Divide/1 -> cosn(si/2)/1
  Constant2/1 -> Divide1/2
  Exponent n Eq: [(1/22.5)*i]+2/1(n) -> Display3/1, Divide1/1
  i/1 -> Exponent n Eq: [(1/22.5)*i]+2/1(i)
  Add/1 -> Divide/2
  Constant1/1 -> Divide/1
  eb.er/1 -> Add/2
  Constant/1 -> Add/1
  Unit Vector/1(Unit Vector) -> eb.er/2
  r/1 -> Embedded MATLAB Function/2(r), Unit Vector/1(Vector)

== system aausat3_lib/Disturbances/Gravity Gradient Torque/  ==
  q(C->SC) : Inport
  "q(I -> SC)" : Inport  Port=2
  R_sc(I) : Inport  Port=3
  Quaternion inverter : aausat3_lib/Math Utilities/Quaternion operations/Quaternion inverter
  Rotation of q1 by q2 : aausat3_lib/Math Utilities/Quaternion operations/Rotation of q1 by q2
  To unit vector : aausat3_lib/Math Utilities/Vector operations/To unit vector
  Vector rotation by q : aausat3_lib/Math Utilities/Quaternion operations/Vector rotation by q
  R_sc(C) : Outport
  wires:
  "q(I -> SC)"/1 -> Rotation of q1 by q2/1
  q(C->SC)/1 -> Quaternion inverter/1
  Quaternion inverter/1 -> Rotation of q1 by q2/2
  R_sc(I)/1 -> To unit vector/1
  Rotation of q1 by q2/1 -> Vector rotation by q/1
  To unit vector/1 -> Vector rotation by q/2
  Vector rotation by q/1 -> R_sc(C)/1

== system aausat3_lib/Math Utilities/Quaternion operations/Quaternion inverter ==
  q : Inport
  Demux : Demux
  Demux1 : Demux  Outputs=3
  Gain : Gain  Gain=-1  SaturateOnIntegerOverflow=on  OutDataTypeStr=Inherit: Same as input  ParamDataTypeStr=Inherit: Same as input
  Mux : Mux
  Mux1 : Mux  Inputs=3
  q^-1 : Outport
  wires:
  q/1 -> Demux/1
  Mux/1 -> q^-1/1
  Demux/4 -> Mux/4
  Demux/1 -> Mux1/1
  Demux/2 -> Mux1/2
  Demux/3 -> Mux1/3
  Mux1/1 -> Gain/1
  Demux1/1 -> Mux/1
  Demux1/2 -> Mux/2
  Demux1/3 -> Mux/3
  Gain/1 -> Demux1/1

== system aausat3_lib/Math Utilities/Quaternion operations/Rotation from q1 to q2 ==
  q1 : Inport
  q2 : Inport  Port=2
  Demux : Demux
  MATLAB Function : MATLAB Function  TreatAsAtomicUnit=on
  Mux : Mux  Inputs=2
  Mux1 : Mux
  Quaternion inverter : Subsystem
  q_diff : Outport
  wires:
  Demux/4 -> Mux1/3
  Demux/3 -> Mux1/2
  Demux/2 -> Mux1/1
  Demux/1 -> Mux1/4
  MATLAB Function/1(y) -> Demux/1
  Mux/1 -> MATLAB Function/1(u)
  q2/1 -> Mux/2
  Mux1/1 -> q_diff/1
  Quaternion inverter/1(q^-1) -> Mux/1
  q1/1 -> Quaternion inverter/1(q)

== system aausat3_lib/Math Utilities/Quaternion operations/Rotation of q1 by q2 ==
  q1 : Inport
  q2 : Inport  Port=2
  Quaternion mulitiplication : S-Function  FunctionName=qmul  EnableBusSupport=off
  q_res : Outport
  wires:
  Quaternion mulitiplication/1 -> q_res/1
  q2/1 -> Quaternion mulitiplication/2
  q1/1 -> Quaternion mulitiplication/1

== system aausat3_lib/Math Utilities/Quaternion operations/Vector rotation by q ==
  q : Inport
  V : Inport  Port=2
  Constant : Constant  Value=0
  Demux : Demux  Outputs=3
  Demux1 : Demux
  Mux : Mux
  Mux1 : Mux  Inputs=3
  Quaternion inverter : Subsystem
  Quaternion mulitiplication : S-Function  FunctionName=qmul  EnableBusSupport=off
  Quaternion mulitiplication1 : S-Function  FunctionName=qmul  EnableBusSupport=off
  Terminator : Terminator
  Vector Concatenate : Concatenate  NumInputs=3
  q'Vq : Outport
  q'Vq_vec : Outport  Port=2
  wires:
  Vector Concatenate/1 -> q'Vq_vec/1
  Demux1/1 -> Vector Concatenate/1, Mux1/1
  Demux1/2 -> Vector Concatenate/2, Mux1/2
  Demux1/3 -> Vector Concatenate/3, Mux1/3
  Demux1/4 -> Terminator/1
  Mux1/1 -> q'Vq/1
  Quaternion inverter/1(q^-1) -> Quaternion mulitiplication/1
  Quaternion mulitiplication/1 -> Quaternion mulitiplication1/1
  q/1 -> Quaternion mulitiplication1/2, Quaternion inverter/1(q)
  V/1 -> Demux/1
  Demux/1 -> Mux/1
  Demux/2 -> Mux/2
  Demux/3 -> Mux/3
  Constant/1 -> Mux/4
  Mux/1 -> Quaternion mulitiplication/2
  Quaternion mulitiplication1/1 -> Demux1/1

== system aausat3_lib/Math Utilities/Quaternion operations/euler2quaternion ==
  Euler angles : Inport
  Mux : Mux
  q1 : Fcn  Expr=sin(u(3)/2)*sin(u(2)/2)*cos(u(1)/2)+cos(u(3)/2)*cos(u(2)/2)*cos(u(1)/2)
  q2 : Fcn  Expr=sin(u(3)/2)*cos(u(2)/2)*cos(u(1)/2)+cos(u(3)/2)*sin(u(2)/2)*sin(u(1)/2)
  q3 : Fcn  Expr=cos(u(3)/2)*sin(u(2)/2)*cos(u(1)/2)+sin(u(3)/2)*cos(u(2)/2)*sin(u(1)/2)
  q4 : Fcn  Expr=cos(u(3)/2)*cos(u(2)/2)*cos(u(1)/2)+sin(u(3)/2)*sin(u(2)/2)*sin(u(1)/2)
  Quaternion : Outport
  wires:
  Mux/1 -> Quaternion/1
  Euler angles/1 -> q1/1, q2/1, q3/1, q4/1
  q3/1 -> Mux/3
  q2/1 -> Mux/2
  q1/1 -> Mux/1
  q4/1 -> Mux/4

== system aausat3_lib/Math Utilities/Quaternion operations/quaternion composition ==
  vector : Inport
  angle : Inport  Port=2
  Demux : Demux  Outputs=3
  Gain : Gain  Gain=1/2  SaturateOnIntegerOverflow=on  OutDataTypeStr=Inherit: Same as input  ParamDataTypeStr=Inherit: Same as input
  Mux : Mux
  Product : Product  SaturateOnIntegerOverflow=on  OutDataTypeStr=Inherit: Same as first input
  Trigonometric Function : Trigonometry  Operator=cos
  Trigonometric Function1 : Trigonometry
  to unit vector : Subsystem
  q : Outport
  wires:
  Mux/1 -> q/1
  Trigonometric Function/1 -> Mux/4
  Demux/3 -> Mux/3
  Demux/2 -> Mux/2
  Demux/1 -> Mux/1
  Product/1 -> Demux/1
  Trigonometric Function1/1 -> Product/2
  to unit vector/1(v_hat) -> Product/1
  vector/1 -> to unit vector/1("v  ")
  Gain/1 -> Trigonometric Function1/1, Trigonometric Function/1
  angle/1 -> Gain/1

== system aausat3_lib/Math Utilities/Quaternion operations/quaternion decomposition ==
  q_in : Inport
  Demux : Demux
  Gain : Gain  Gain=2  SaturateOnIntegerOverflow=on  OutDataTypeStr=Inherit: Same as input  ParamDataTypeStr=Inherit: Same as input
  Math Function : Math  Operator=reciprocal  SaturateOnIntegerOverflow=on
  Mux : Mux  Inputs=3
  Product : Product  SaturateOnIntegerOverflow=on  OutDataTypeStr=Inherit: Same as first input
  Trigonometric Function : Trigonometry  Operator=acos
  Trigonometric Function1 : Trigonometry
  to unit vector : Subsystem
  Vector : Outport
  Angle : Outport  Port=2
  wires:
  to unit vector/1(v_hat) -> Vector/1
  Product/1 -> to unit vector/1("v  ")
  Trigonometric Function1/1 -> Math Function/1
  Math Function/1 -> Product/2
  Mux/1 -> Product/1
  Demux/3 -> Mux/3
  Demux/2 -> Mux/2
  Demux/1 -> Mux/1
  Gain/1 -> Angle/1
  Trigonometric Function/1 -> Trigonometric Function1/1, Gain/1
  Demux/4 -> Trigonometric Function/1
  q_in/1 -> Demux/1

== system aausat3_lib/Math Utilities/Quaternion operations/quaternion2euler ==
  quaternion : Inport
  Mux : Mux  Inputs=3
  theta 1 : Fcn  Expr=-atan2((2*(u(2)*u(3) + u(1)*u(4))),(1-2*(u(1)*u(1) + u(2)*u(2))))
  theta 2 : Fcn  Expr=-asin(2*(u(1)*u(3)-u(2)*u(4)))
  theta 3 : Fcn  Expr=-atan2((2*(u(1)*u(2) + u(3)*u(4))),(1-2*(u(2)*u(2) + u(3)*u(3))))
  Euler angles : Outport
  wires:
  theta 1/1 -> Mux/1
  theta 2/1 -> Mux/2
  theta 3/1 -> Mux/3
  quaternion/1 -> theta 2/1, theta 1/1, theta 3/1
  Mux/1 -> Euler angles/1

== system aausat3_lib/Math Utilities/Quaternion operations/w to q ==
  Angular velocity : Inport
  Initial quaternion : Inport  Port=2
  S-Function : S-Function  FunctionName=qestimator  EnableBusSupport=off
  estimated quaternion : Outport
  wires:
  Angular velocity/1 -> S-Function/2
  Initial quaternion/1 -> S-Function/1
  S-Function/1 -> estimated quaternion/1

== system aausat3_lib/Math Utilities/Vector operations/Cross Product ==
  v : Inport
  u : Inport  Port=2
  Demux : Demux  Outputs=3
  Demux1 : Demux  Outputs=3
  Mux : Mux  Inputs=3
  Product{1..6} (6 alike) : Product  SaturateOnIntegerOverflow=on  OutDataTypeStr=Inherit: Same as first input
  Sum : Sum  Inputs=-+|
  Sum1 : Sum  Inputs=-+|
  Sum2 : Sum  Inputs=-+|
  v x u : Outport
  wires:
  v/1 -> Demux1/1
  u/1 -> Demux/1
  Product3/1 -> Sum/2
  Product1/1 -> Sum/1
  Product4/1 -> Sum1/2
  Product2/1 -> Sum1/1
  Product6/1 -> Sum2/2
  Product5/1 -> Sum2/1
  Demux1/2 -> Product3/1, Product5/1
  Demux/3 -> Product3/2, Product2/2
  Demux1/3 -> Product1/1, Product4/1
  Demux/2 -> Product1/2, Product6/2
  Demux/1 -> Product4/2, Product5/2
  Demux1/1 -> Product2/1, Product6/1
  Sum/1 -> Mux/1
  Sum1/1 -> Mux/2
  Sum2/1 -> Mux/3
  Mux/1 -> v x u/1

== system aausat3_lib/Math Utilities/Vector operations/To unit vector ==
  "v  " : Inport
  Constant : Constant
  Dot Product : DotProduct  InputSameDT=on  OutDataTypeStr=Inherit: Inherit via internal rule
  Math Function : Math  Operator=reciprocal  SaturateOnIntegerOverflow=on
  Product : Product  SaturateOnIntegerOverflow=on  OutDataTypeStr=Inherit: Same as first input
  Switch : Switch  Criteria=u2 ~= 0  SaturateOnIntegerOverflow=on
  sqrt : Math  Operator=sqrt  SaturateOnIntegerOverflow=on
  v_hat : Outport
  wires:
  Constant/1 -> Switch/3
  sqrt/1 -> Switch/1, Switch/2
  Switch/1 -> Math Function/1
  "v  "/1 -> Product/1, Dot Product/1, Dot Product/2
  Math Function/1 -> Product/2
  Product/1 -> v_hat/1
  Dot Product/1 -> sqrt/1

== system aausat3_lib/On-board Software/Ephemeris/ECI->ECEF quaternion ==
  t(JD) : Inport
  eci2ecef : MATLABFcn  MATLABFcn=eci2ecef  OutputDimensions=4
  q(I->E) : Outport
  wires:
  eci2ecef/1 -> q(I->E)/1
  t(JD)/1 -> eci2ecef/1

== system aausat3_lib/On-board Software/Ephemeris/Sun Position ==
  t(JD) : Inport
  Sun R in ECI : MATLABFcn  MATLABFcn=sun  OutputDimensions=3
  R_s(I) : Outport
  wires:
  t(JD)/1 -> Sun R in ECI/1
  Sun R in ECI/1 -> R_s(I)/1

== system aausat3_lib/On-board Software/Orbit and Magnetic field models/(IGRF) Magnetic field ==
  Spacecraft position R_sc(I) : Inport
  Earth rotation q(I->E) : Inport  Port=2
  Enable : EnablePort
  Magnetic field model : Subsystem
  T->Gauss : Gain  Gain=1e4  SaturateOnIntegerOverflow=on  OutDataTypeStr=Inherit: Same as input  ParamDataTypeStr=Inherit: Same as input
  Vector rotation by q : Subsystem
  Magnetic field vector B(E) : Outport
  wires:
  T->Gauss/1 -> Magnetic field vector B(E)/1
  Magnetic field model/1(B(E)) -> T->Gauss/1  "B(I / E)"
  Vector rotation by q/1(q'Vq) -> Magnetic field model/1(R_sc(E))
  Earth rotation q(I->E)/1 -> Vector rotation by q/1(q)
  Spacecraft position R_sc(I)/1 -> Vector rotation by q/2(V)

== system aausat3_lib/On-board Software/Orbit and Magnetic field models/Custom time ==
  Initial time ti(JD) : Inport
  Enable : EnablePort
  Clock : Clock
  Sec2Day : Gain  Gain=1/86400  SaturateOnIntegerOverflow=on  OutDataTypeStr=Inherit: Same as input  ParamDataTypeStr=Inherit: Same as input
  Sum : Sum  Inputs=|++
  Simulation time t(JD) : Outport
  wires:
  Initial time ti(JD)/1 -> Sum/1
  Sec2Day/1 -> Sum/2
  Clock/1 -> Sec2Day/1
  Sum/1 -> Simulation time t(JD)/1

== system aausat3_lib/On-board Software/Orbit and Magnetic field models/Eclipse model ==
  note: theta_e
  Sun vector (I) : Inport
  Satellite (I) : Inport  Port=2
  Enable : EnablePort
  Constant : Constant  Value=pi
  Constant1 : Constant  Value=enable
  Divide : Product  Inputs=*/
  Dot Product : DotProduct  InputSameDT=on  OutDataTypeStr=Inherit: Inherit via internal rule
  Dot Product1 : DotProduct  InputSameDT=on  OutDataTypeStr=Inherit: Inherit via internal rule
  Earth radius : Constant  Value=r_e
  False : Constant  Value=0
  Math Function : Math  Operator=sqrt  SaturateOnIntegerOverflow=on
  Max angle : Constant  Value=theta_e/180*pi
  Sum : Sum  Inputs=-+|
  Sum1 : Sum  Inputs=+-|
  Switch : Switch
  Switch1 : Switch  Criteria=u2 > Threshold
  To unit vector : Subsystem
  To unit vector1 : Subsystem
  Trigonometric Function : Trigonometry  Operator=asin
  Trigonometric Function1 : Trigonometry  Operator=acos
  True : Constant
  Eclipse : Outport  PortDimensions=1
  wires:
  Max angle/1 -> Switch1/1
  Constant1/1 -> Switch1/2
  Sun vector (I)/1 -> To unit vector/1("v  ")
  Satellite (I)/1 -> To unit vector1/1("v  "), Dot Product1/1, Dot Product1/2
  To unit vector/1(v_hat) -> Dot Product/1
  To unit vector1/1(v_hat) -> Dot Product/2
  Dot Product/1 -> Trigonometric Function1/1
  Earth radius/1 -> Divide/1
  Math Function/1 -> Divide/2
  Divide/1 -> Trigonometric Function/1
  Trigonometric Function1/1 -> Sum/1
  Constant/1 -> Sum/2
  Sum/1 -> Sum1/1  "theta"
  Sum1/1 -> Switch/2
  True/1 -> Switch/3
  False/1 -> Switch/1
  Switch/1 -> Eclipse/1
  Switch1/1 -> Sum1/2
  Trigonometric Function/1 -> Switch1/3
  Dot Product1/1 -> Math Function/1

== system aausat3_lib/On-board Software/Orbit and Magnetic field models/Quaternion inverter ==
  q : Inport
  Demux : Demux
  Demux1 : Demux  Outputs=3
  Gain : Gain  Gain=-1  SaturateOnIntegerOverflow=on  OutDataTypeStr=Inherit: Same as input  ParamDataTypeStr=Inherit: Same as input
  Mux : Mux
  Mux1 : Mux  Inputs=3
  q^-1 : Outport
  wires:
  Gain/1 -> Demux1/1
  Demux1/3 -> Mux/3
  Demux1/2 -> Mux/2
  Demux1/1 -> Mux/1
  Mux1/1 -> Gain/1
  Demux/3 -> Mux1/3
  Demux/2 -> Mux1/2
  Demux/1 -> Mux1/1
  Demux/4 -> Mux/4
  Mux/1 -> q^-1/1
  q/1 -> Demux/1

== system aausat3_lib/On-board Software/Orbit and Magnetic field models/SGP4 position ==
  JD : Inport
  TLE : Inport  Port=2
  Enable : EnablePort
  " S-Function" : S-Function  FunctionName=sgp4S  EnableBusSupport=off
  Demux : Demux  Outputs=12
  Demux1 : Demux  Outputs=[3 3]
  JD to Minutes : Gain  Gain=1440
  Mux : Mux  Inputs=2
  Mux1 : Mux  Inputs=12
  Sum : Sum  Inputs=-+|  SaturateOnIntegerOverflow=on  InputSameDT=on  OutDataTypeStr=Inherit: Same as first input
  "TLE -> JD converter" : Subsystem
  "km -> m" : Gain  Gain=1000  SaturateOnIntegerOverflow=on  OutDataTypeStr=Inherit: Same as input  ParamDataTypeStr=Inherit: Same as input
  "km/s -> m/s" : Gain  Gain=1000  SaturateOnIntegerOverflow=on  OutDataTypeStr=Inherit: Same as input  ParamDataTypeStr=Inherit: Same as input
  Position (I) : Outport  InitialOutput=0
  Velocity (I) : Outport  Port=2  InitialOutput=0
  wires:
  JD to Minutes/1 -> Mux/1
  Sum/1 -> JD to Minutes/1
  "TLE -> JD converter"/1(JD) -> Sum/1, Mux1/1
  Demux/1 -> "TLE -> JD converter"/1(TLE (Epoch time))
  Mux1/1 -> Mux/2
  Demux/12 -> Mux1/12
  Demux/11 -> Mux1/11
  Demux/10 -> Mux1/10
  Demux/9 -> Mux1/9
  Demux/8 -> Mux1/8
  Demux/7 -> Mux1/7
  Demux/6 -> Mux1/6
  Demux/5 -> Mux1/5
  Demux/4 -> Mux1/4
  Demux/3 -> Mux1/3
  Demux/2 -> Mux1/2
  TLE/1 -> Demux/1
  Demux1/1 -> "km -> m"/1
  Demux1/2 -> "km/s -> m/s"/1
  " S-Function"/1 -> Demux1/1
  Mux/1 -> " S-Function"/1
  "km/s -> m/s"/1 -> Velocity (I)/1
  "km -> m"/1 -> Position (I)/1
  JD/1 -> Sum/2

== system aausat3_lib/On-board Software/Orbit and Magnetic field models/Vector rotation by q ==
  q : Inport
  V : Inport  Port=2
  Constant : Constant  Value=0
  Demux : Demux  Outputs=3
  Demux1 : Demux
  Mux : Mux
  Mux1 : Mux  Inputs=3
  Quaternion inverter : Subsystem
  Quaternion mulitiplication : S-Function  FunctionName=qmul  EnableBusSupport=off
  Quaternion mulitiplication1 : S-Function  FunctionName=qmul  EnableBusSupport=off
  Terminator : Terminator
  q'Vq : Outport
  wires:
  Mux1/1 -> q'Vq/1
  Demux1/4 -> Terminator/1
  Demux1/3 -> Mux1/3
  Demux1/2 -> Mux1/2
  Demux1/1 -> Mux1/1
  Quaternion mulitiplication1/1 -> Demux1/1
  Quaternion mulitiplication/1 -> Quaternion mulitiplication1/1
  Mux/1 -> Quaternion mulitiplication/2
  Constant/1 -> Mux/4
  Demux/3 -> Mux/3
  Demux/2 -> Mux/2
  Demux/1 -> Mux/1
  V/1 -> Demux/1
  Quaternion inverter/1(q^-1) -> Quaternion mulitiplication/1
  q/1 -> Quaternion mulitiplication1/2, Quaternion inverter/1(q)
